simulink model "ba"  (R2022a)
settings: Solver=ode45  StartTime=0.0  StopTime=20  FixedStep=0.001  MaxStep=0.4  RelTol=1e-3  EnableMultiTasking=on
settings Model: ExtModeTrigMode=oneshot  ExtModeArmWhenConnect=off  Creator=liujk  LastModifiedBy=961007prl
settings SolverCC: AlgebraicLoopSolver=TrustRegion
settings DataIOCC: SaveFormat=Array  SignalLoggingSaveFormat=ModelDataLogs  ReturnWorkspaceOutputs=off  SignalLoggingName=sigsOut
settings OptimizationCC: BooleanDataType=off  LifeSpan=inf
settings DebuggingCC: SaveWithParameterizedLinksMsg=none  UnderspecifiedInitializationDetection=Classic  MergeDetectMultiDrivingBlocksExec=none  SignalResolutionControl=TryResolveAllWithWarning  MultiTaskDSMMsg=warning  MultiTaskCondExecSysMsg=none  UnconnectedInputMsg=warning  UnconnectedOutputMsg=warning  UnconnectedLineMsg=warning  StateNameClashWarn=warning  SFUnexpectedBacktrackingDiag=warning  SFNoUnconditionalDefaultTransitionDiag=warning  SFExecutionAtInitializationDiag=none  SFMachineParentedDataDiag=warning  ArithmeticOperatorsInVariantConditions=warning
settings HardwareCC: ProdBitPerPointer=32  ProdBitPerSizeT=32  ProdBitPerPtrDiffT=32  ProdLargestAtomicFloat=None  ProdIntDivRoundTo=Undefined  ProdEndianess=Unspecified  ProdWordSize=32  ProdHWDeviceType=32-bit Generic  TargetUnknown=on
settings ModelReferenceCC: PropagateSignalLabelsOutOfModel=off
settings SFSimCC: SimUseLocalCustomCode=off  CustomCodeUndefinedFunction=UseInterfaceOnly
settings RTWCC: RTWUseLocalCustomCode=off
settings CodeAppCC: StateflowObjectComments=on
settings GRTTargetCC: TargetLangStandard=C89/C90 (ANSI)  CombineOutputUpdateFcns=off  GRTInterface=on
settings ConfigComp: CovMetricSettings=dw  CovSaveCumulativeToWorkspaceVar=on  CovSaveSingleToWorkspaceVar=on  CovExternalEMLEnable=off  CovSFcnEnable=off

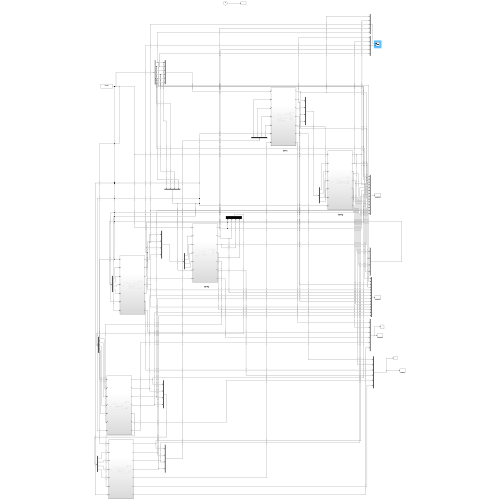
[thumbnail: Simulink's stored preview of the top-level diagram]
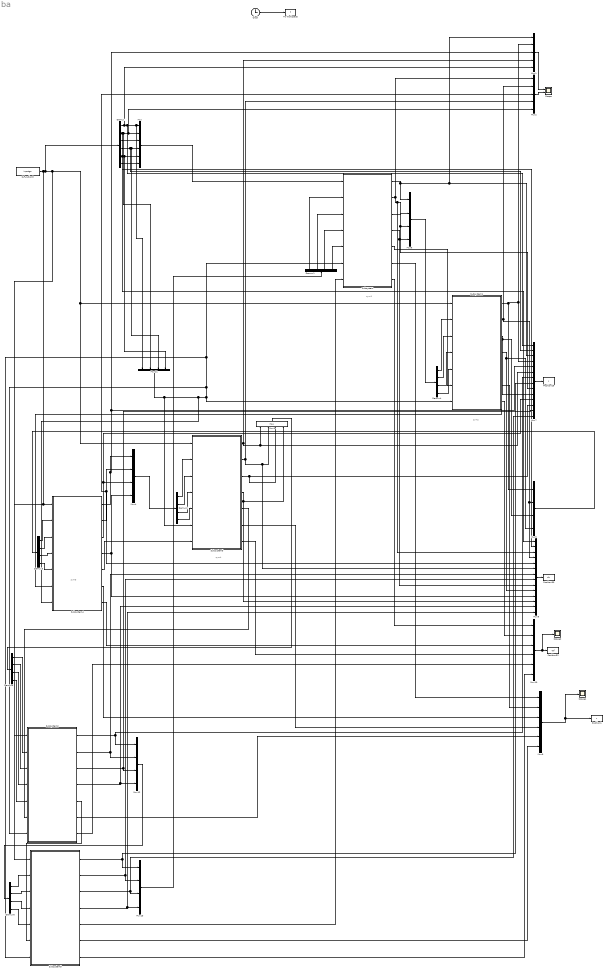
== system ba ==
  note: sym3
  note: sym4
  note: sym2
  note: sym1
  Clock : Clock
  Demux : Demux  Outputs=6
  Demux{1..6} (6 alike) : Demux
  Mux : Mux  Inputs=6
  Mux1 : Mux  Inputs=5
  Mux10 : Mux  Inputs=6
  Mux{3..6,11..13} (7 alike) : Mux
  Mux2 : Mux  Inputs=5
  Mux7 : Mux  Inputs=14
  Mux8 : Mux  Inputs=14
  Mux9 : Mux  Inputs=6
  Position1 : ToWorkspace  VariableName=v  SampleTime=-1
  Position29 : ToWorkspace  VariableName=x  SampleTime=-1
  Position30 : ToWorkspace  VariableName=dx  SampleTime=-1
  Position32 : ToWorkspace  VariableName=Wf  SampleTime=-1
  S-Function3 : S-Function  FunctionName=inputgc  SFunctionDeploymentMode=off  EnableBusSupport=off
  Scope : Scope  NumInputPorts=2
  Scope1 : Scope
  Scope2 : Scope
  Subsystem : Subsystem
  Subsystem1 : Subsystem
  Subsystem2 : Subsystem
  Subsystem3 : Subsystem
  Subsystem4 : Subsystem
  Subsystem5 : Subsystem
  To Workspace : ToWorkspace  VariableName=t  SampleTime=-1
  wires:
  Subsystem/1(Out1) -> Mux6/1, Mux7/3, Mux1/1
  Subsystem/3(Out6) -> Mux7/9, Mux6/3
  Subsystem1/4(Out7) -> Mux8/10, Mux5/4
  Subsystem1/2(Out5) -> Mux5/2, Mux8/4, Mux2/2
  Subsystem4/4(Out7) -> Mux8/11, Mux4/4
  Subsystem4/3(Out6) -> Mux7/11, Mux4/3
  Subsystem4/2(Out5) -> Mux2/3, Mux4/2, Mux8/5
  Subsystem3/1(Out1) -> Mux7/6, Mux3/1, Mux1/4
  Subsystem3/3(Out6) -> Mux3/3, Mux7/12
  S-Function3/1 -> Subsystem5/1(In2), Subsystem3/1(In2), Subsystem1/1(In2), Demux/1, Subsystem2/1(In2), Subsystem4/1(In2)
  Demux/2 -> Mux2/5, Mux/2, Mux11/2, Mux8/1
  Demux/5 -> Mux/5, Mux11/4, Mux8/2
  Subsystem1/7(Out2) -> Mux10/2
  Subsystem/7(Out2) -> Mux10/1
  Demux/6 -> Mux/6
  Demux/4 -> Mux11/3, Mux/4, Mux7/2
  Mux2/1 -> Scope/2
  Mux7/1 -> Position29/1
  Subsystem/4(Out7) -> Mux8/9, Mux6/4
  Demux/3 -> Mux/3
  Subsystem4/7(Out2) -> Mux10/3
  Subsystem4/1(Out1) -> Mux4/1, Mux7/5, Mux1/3
  Mux10/1 -> Scope2/1, Position32/1
  Subsystem1/3(Out6) -> Mux7/10, Mux5/3
  Demux1/1 -> Subsystem/2(In2)
  Demux2/1 -> Subsystem3/2(In1)
  Subsystem3/7(Out2) -> Mux10/4
  Demux2/3 -> Subsystem3/4(In8)
  Demux1/4 -> Subsystem/5(In5)
  Demux3/2 -> Subsystem4/3(In4)
  Demux2/2 -> Subsystem3/3(In7)
  Mux1/1 -> Scope/1
  Clock/1 -> To Workspace/1
  Demux3/4 -> Subsystem4/5(In6)
  Demux3/1 -> Subsystem4/2(In3)
  Subsystem1/1(Out1) -> Mux5/1, Mux7/4, Mux1/2
  Demux3/3 -> Subsystem4/4(In5)
  Mux/1 -> Subsystem/1(In1)
  Demux4/2 -> Subsystem1/3(In4)
  Subsystem/2(Out5) -> Mux8/3, Mux6/2, Mux2/1
  Subsystem3/4(Out7) -> Mux8/12, Mux3/4
  Demux1/2 -> Subsystem/3(In3)
  Mux8/1 -> Position30/1
  Demux1/3 -> Subsystem/4(In4)
  Demux4/3 -> Subsystem1/4(In5)
  Demux4/4 -> Subsystem1/5(In6)
  Demux/1 -> Mux/1, Mux11/1, Mux7/1, Mux1/5
  Demux4/1 -> Subsystem1/2(In3)
  Subsystem3/2(Out5) -> Mux8/6, Mux3/2, Mux2/4
  Demux2/4 -> Subsystem3/5(In9)
  Mux5/1 -> Demux3/1
  Mux11/1 -> Subsystem4/7(In7), Subsystem5/7(In7), Subsystem/6(In6), Subsystem2/7(In7), Subsystem1/7(In7), Subsystem3/6(In10)
  Mux6/1 -> Demux4/1
  Subsystem/5(Out3) -> Subsystem1/6(In1)
  Subsystem1/5(Out3) -> Subsystem4/6(In1)
  Mux9/1 -> Scope1/1, Position1/1
  Subsystem/6(Out4) -> Mux9/1
  Subsystem1/6(Out4) -> Mux9/2
  Subsystem4/6(Out4) -> Mux9/3
  Subsystem3/6(Out4) -> Mux9/4
  Demux5/1 -> Subsystem2/2(In3)
  Demux5/2 -> Subsystem2/3(In4)
  Demux5/3 -> Subsystem2/4(In5)
  Demux5/4 -> Subsystem2/5(In6)
  Subsystem2/3(Out6) -> Mux12/3, Mux7/13
  Subsystem2/4(Out7) -> Mux8/13, Mux12/4
  Subsystem2/1(Out1) -> Mux12/1, Mux7/7
  Subsystem2/2(Out5) -> Mux12/2, Mux8/7
  Subsystem5/2(Out5) -> Mux13/2, Mux8/8
  Subsystem5/3(Out6) -> Mux13/3, Mux7/14
  Subsystem5/4(Out7) -> Mux8/14, Mux13/4
  Subsystem5/1(Out1) -> Mux13/1, Mux7/8
  Demux6/1 -> Subsystem5/2(In3)
  Demux6/2 -> Subsystem5/3(In4)
  Demux6/3 -> Subsystem5/4(In5)
  Demux6/4 -> Subsystem5/5(In6)
  Mux12/1 -> Demux6/1
  Subsystem2/5(Out3) -> Subsystem5/6(In1)
  Subsystem2/6(Out4) -> Mux9/5
  Subsystem5/6(Out4) -> Mux9/6
  Subsystem5/5(Out3) -> Subsystem/7(In7)
  Subsystem4/5(Out3) -> Subsystem3/7(In3)
  Subsystem3/5(Out3) -> Subsystem2/6(In1)
  Mux13/1 -> Demux1/1
  Mux3/1 -> Demux5/1
  Subsystem2/7(Out2) -> Mux10/5
  Subsystem5/7(Out2) -> Mux10/6
  Mux4/1 -> Demux2/1

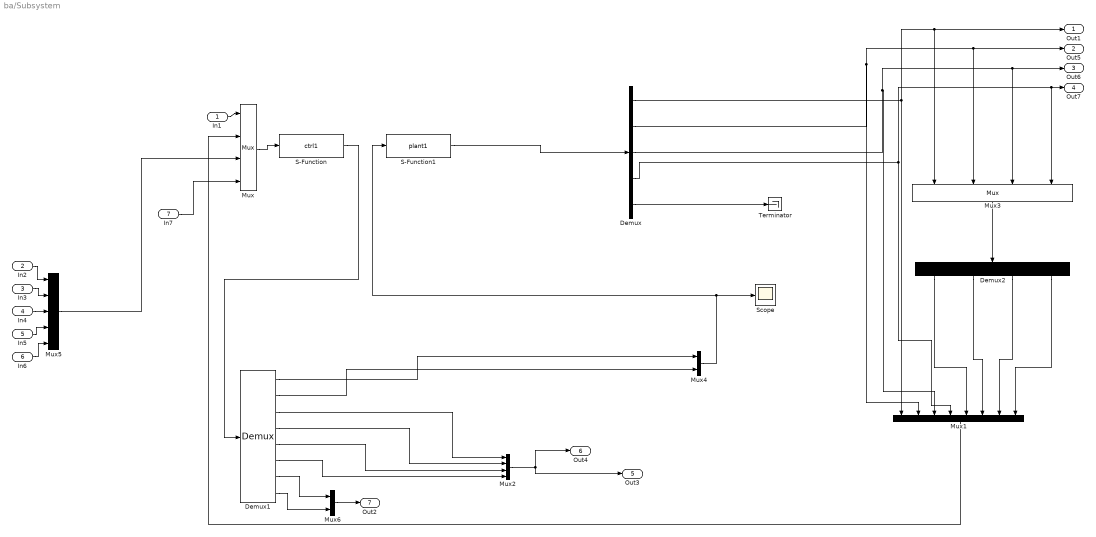
== system ba/Subsystem ==
  In1 : Inport
  In2 : Inport  Port=2
  In3 : Inport  Port=3
  In4 : Inport  Port=4
  In5 : Inport  Port=5
  In6 : Inport  Port=6
  In7 : Inport  Port=7
  Demux : Demux  Outputs=5
  Demux1 : Demux  Outputs=8
  Demux2 : Demux
  Mux : Mux
  Mux1 : Mux  Inputs=8
  Mux2 : Mux
  Mux3 : Mux
  Mux4 : Mux  Inputs=2
  Mux5 : Mux  Inputs=5
  Mux6 : Mux  Inputs=2
  S-Function : S-Function  FunctionName=ctrl1  SFunctionDeploymentMode=off  EnableBusSupport=off
  S-Function1 : S-Function  FunctionName=plant1  SFunctionDeploymentMode=off  EnableBusSupport=off
  Scope : Scope
  Terminator : Terminator
  Out1 : Outport
  Out5 : Outport  Port=2
  Out6 : Outport  Port=3
  Out7 : Outport  Port=4
  Out3 : Outport  Port=5
  Out4 : Outport  Port=6
  Out2 : Outport  Port=7
  wires:
  Mux/1 -> S-Function/1
  In1/1 -> Mux/1
  S-Function/1 -> Demux1/1
  Demux1/1 -> Mux4/1
  Mux4/1 -> S-Function1/1, Scope/1
  S-Function1/1 -> Demux/1
  Demux/5 -> Terminator/1
  Demux1/2 -> Mux4/2
  In2/1 -> Mux5/1
  In3/1 -> Mux5/2
  In4/1 -> Mux5/3
  In5/1 -> Mux5/4
  In6/1 -> Mux5/5
  Mux5/1 -> Mux/3
  Mux1/1 -> Mux/2
  Demux/2 -> Mux3/2, Out5/1, Mux1/2
  Demux2/3 -> Mux1/7
  Demux2/4 -> Mux1/8
  Demux2/2 -> Mux1/6
  Demux/3 -> Mux3/3, Out6/1, Mux1/3
  Demux/4 -> Mux3/4, Out7/1, Mux1/4
  Demux/1 -> Mux3/1, Out1/1, Mux1/1
  Demux2/1 -> Mux1/5
  Demux1/3 -> Mux2/1
  Demux1/4 -> Mux2/2
  Demux1/5 -> Mux2/3
  Demux1/6 -> Mux2/4
  Mux2/1 -> Out3/1, Out4/1
  In7/1 -> Mux/4
  Demux1/7 -> Mux6/1
  Demux1/8 -> Mux6/2
  Mux6/1 -> Out2/1
  Mux3/1 -> Demux2/1

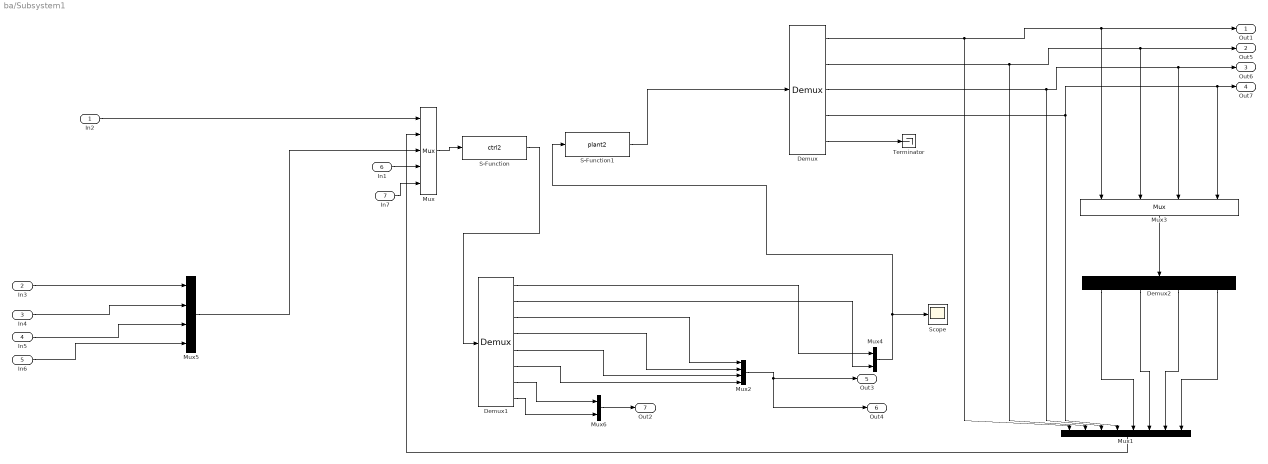
== system ba/Subsystem1 ==
  In2 : Inport
  In3 : Inport  Port=2
  In4 : Inport  Port=3
  In5 : Inport  Port=4
  In6 : Inport  Port=5
  In1 : Inport  Port=6
  In7 : Inport  Port=7
  Demux : Demux  Outputs=5
  Demux1 : Demux  Outputs=8
  Demux2 : Demux
  Mux : Mux  Inputs=5
  Mux1 : Mux  Inputs=8
  Mux2 : Mux
  Mux3 : Mux
  Mux4 : Mux  Inputs=2
  Mux5 : Mux
  Mux6 : Mux  Inputs=2
  S-Function : S-Function  FunctionName=ctrl2  SFunctionDeploymentMode=off  EnableBusSupport=off
  S-Function1 : S-Function  FunctionName=plant2  SFunctionDeploymentMode=off  EnableBusSupport=off
  Scope : Scope
  Terminator : Terminator
  Out1 : Outport
  Out5 : Outport  Port=2
  Out6 : Outport  Port=3
  Out7 : Outport  Port=4
  Out3 : Outport  Port=5
  Out4 : Outport  Port=6
  Out2 : Outport  Port=7
  wires:
  Mux/1 -> S-Function/1
  S-Function/1 -> Demux1/1
  Demux1/1 -> Mux4/1
  S-Function1/1 -> Demux/1
  Demux/5 -> Terminator/1
  In3/1 -> Mux5/1
  In4/1 -> Mux5/2
  In5/1 -> Mux5/3
  In6/1 -> Mux5/4
  In2/1 -> Mux/1
  Mux5/1 -> Mux/3
  Mux4/1 -> S-Function1/1, Scope/1
  Demux2/3 -> Mux1/7
  Demux/1 -> Out1/1, Mux3/1, Mux1/1
  Demux2/2 -> Mux1/6
  Mux1/1 -> Mux/2
  Demux2/1 -> Mux1/5
  Demux/2 -> Out5/1, Mux3/2, Mux1/2
  Demux2/4 -> Mux1/8
  Demux/3 -> Out6/1, Mux3/3, Mux1/3
  Demux/4 -> Out7/1, Mux3/4, Mux1/4
  Mux3/1 -> Demux2/1
  Demux1/2 -> Mux4/2
  Demux1/4 -> Mux2/2
  Mux2/1 -> Out3/1, Out4/1
  Demux1/3 -> Mux2/1
  Demux1/5 -> Mux2/3
  Demux1/6 -> Mux2/4
  In1/1 -> Mux/4
  In7/1 -> Mux/5
  Demux1/7 -> Mux6/1
  Demux1/8 -> Mux6/2
  Mux6/1 -> Out2/1

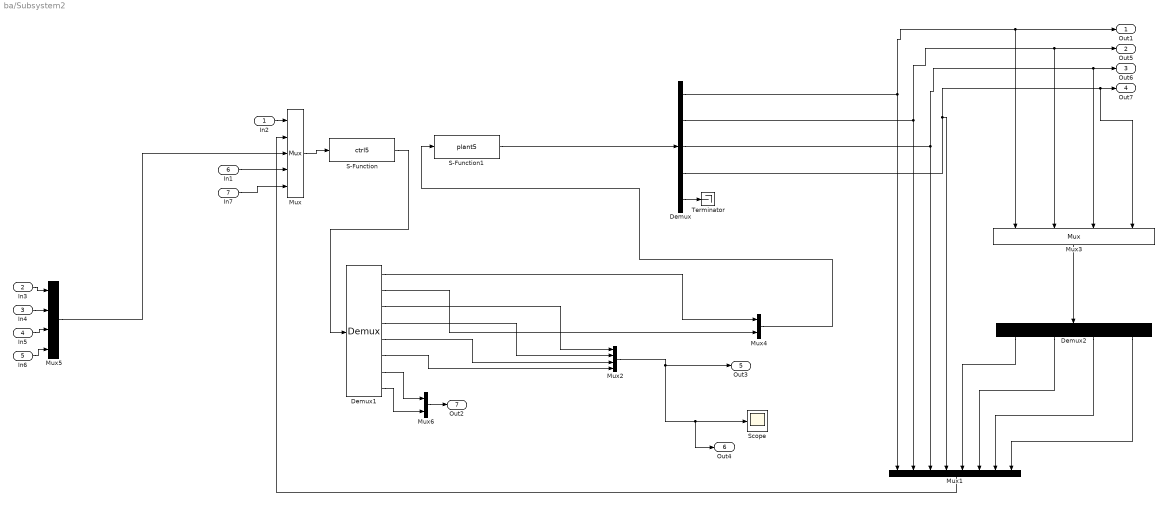
== system ba/Subsystem2 ==
  In2 : Inport
  In3 : Inport  Port=2
  In4 : Inport  Port=3
  In5 : Inport  Port=4
  In6 : Inport  Port=5
  In1 : Inport  Port=6
  In7 : Inport  Port=7
  Demux : Demux  Outputs=5
  Demux1 : Demux  Outputs=8
  Demux2 : Demux
  Mux : Mux  Inputs=5
  Mux1 : Mux  Inputs=8
  Mux2 : Mux
  Mux3 : Mux
  Mux4 : Mux  Inputs=2
  Mux5 : Mux
  Mux6 : Mux  Inputs=2
  S-Function : S-Function  FunctionName=ctrl5  SFunctionDeploymentMode=off  EnableBusSupport=off
  S-Function1 : S-Function  FunctionName=plant5  SFunctionDeploymentMode=off  EnableBusSupport=off
  Scope : Scope
  Terminator : Terminator
  Out1 : Outport
  Out5 : Outport  Port=2
  Out6 : Outport  Port=3
  Out7 : Outport  Port=4
  Out3 : Outport  Port=5
  Out4 : Outport  Port=6
  Out2 : Outport  Port=7
  wires:
  Mux/1 -> S-Function/1
  S-Function/1 -> Demux1/1
  S-Function1/1 -> Demux/1
  Demux/5 -> Terminator/1
  In3/1 -> Mux5/1
  In4/1 -> Mux5/2
  In5/1 -> Mux5/3
  In6/1 -> Mux5/4
  In2/1 -> Mux/1
  Mux5/1 -> Mux/3
  Mux4/1 -> S-Function1/1
  Mux1/1 -> Mux/2
  Demux1/1 -> Mux4/1
  Demux1/2 -> Mux4/2
  Demux/2 -> Out5/1, Mux3/2, Mux1/2
  Demux2/3 -> Mux1/7
  Demux2/4 -> Mux1/8
  Demux2/2 -> Mux1/6
  Demux/3 -> Out6/1, Mux3/3, Mux1/3
  Demux/4 -> Out7/1, Mux3/4, Mux1/4
  Demux/1 -> Mux3/1, Out1/1, Mux1/1
  Demux2/1 -> Mux1/5
  Mux3/1 -> Demux2/1
  Demux1/4 -> Mux2/2
  Mux2/1 -> Out3/1, Out4/1, Scope/1
  Demux1/3 -> Mux2/1
  Demux1/5 -> Mux2/3
  Demux1/6 -> Mux2/4
  In1/1 -> Mux/4
  In7/1 -> Mux/5
  Demux1/7 -> Mux6/1
  Demux1/8 -> Mux6/2
  Mux6/1 -> Out2/1

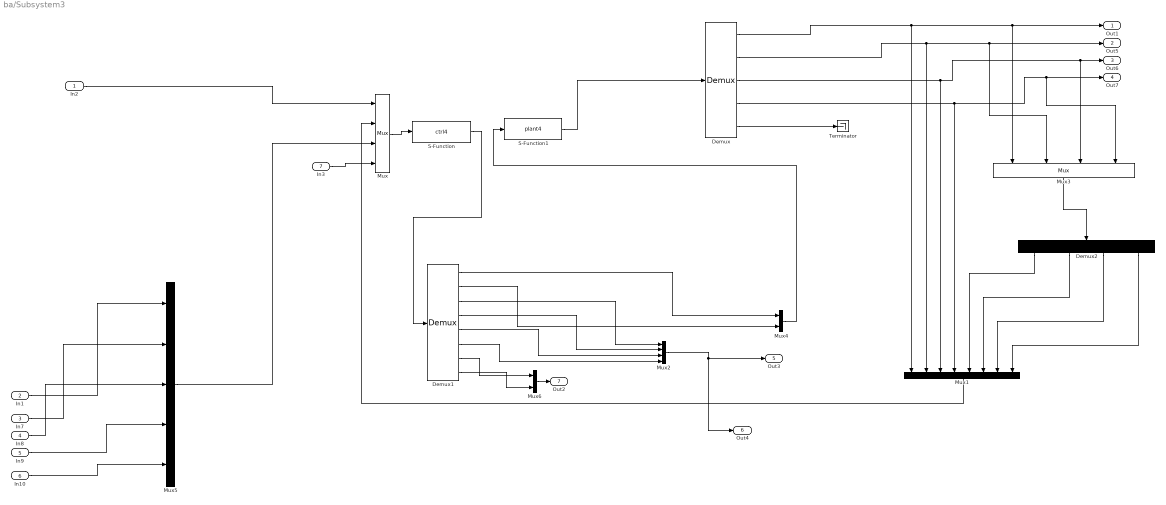
== system ba/Subsystem3 ==
  In2 : Inport
  In1 : Inport  Port=2
  In7 : Inport  Port=3
  In8 : Inport  Port=4
  In9 : Inport  Port=5
  In10 : Inport  Port=6
  In3 : Inport  Port=7
  Demux : Demux  Outputs=5
  Demux1 : Demux  Outputs=8
  Demux2 : Demux
  Mux : Mux
  Mux1 : Mux  Inputs=8
  Mux2 : Mux
  Mux3 : Mux
  Mux4 : Mux  Inputs=2
  Mux5 : Mux  Inputs=5
  Mux6 : Mux  Inputs=2
  S-Function : S-Function  FunctionName=ctrl4  SFunctionDeploymentMode=off  EnableBusSupport=off
  S-Function1 : S-Function  FunctionName=plant4  SFunctionDeploymentMode=off  EnableBusSupport=off
  Terminator : Terminator
  Out1 : Outport
  Out5 : Outport  Port=2
  Out6 : Outport  Port=3
  Out7 : Outport  Port=4
  Out3 : Outport  Port=5
  Out4 : Outport  Port=6
  Out2 : Outport  Port=7
  wires:
  Mux/1 -> S-Function/1
  S-Function/1 -> Demux1/1
  Demux1/1 -> Mux4/1
  S-Function1/1 -> Demux/1
  Demux/5 -> Terminator/1
  In2/1 -> Mux/1
  Mux5/1 -> Mux/3
  Mux4/1 -> S-Function1/1
  In1/1 -> Mux5/1
  In7/1 -> Mux5/2
  In8/1 -> Mux5/3
  In9/1 -> Mux5/4
  In10/1 -> Mux5/5
  Mux1/1 -> Mux/2
  Demux/2 -> Mux3/2, Out5/1, Mux1/2
  Demux2/3 -> Mux1/7
  Demux2/4 -> Mux1/8
  Demux2/2 -> Mux1/6
  Demux/3 -> Mux1/3, Mux3/3, Out6/1
  Demux/4 -> Mux1/4, Mux3/4, Out7/1
  Demux/1 -> Mux1/1, Mux3/1, Out1/1
  Demux2/1 -> Mux1/5
  Demux1/2 -> Mux4/2
  Demux1/4 -> Mux2/2
  Demux1/3 -> Mux2/1
  Demux1/5 -> Mux2/3
  Demux1/6 -> Mux2/4
  In3/1 -> Mux/4
  Mux2/1 -> Out3/1, Out4/1
  Demux1/7 -> Mux6/1
  Demux1/8 -> Mux6/2
  Mux6/1 -> Out2/1
  Mux3/1 -> Demux2/1

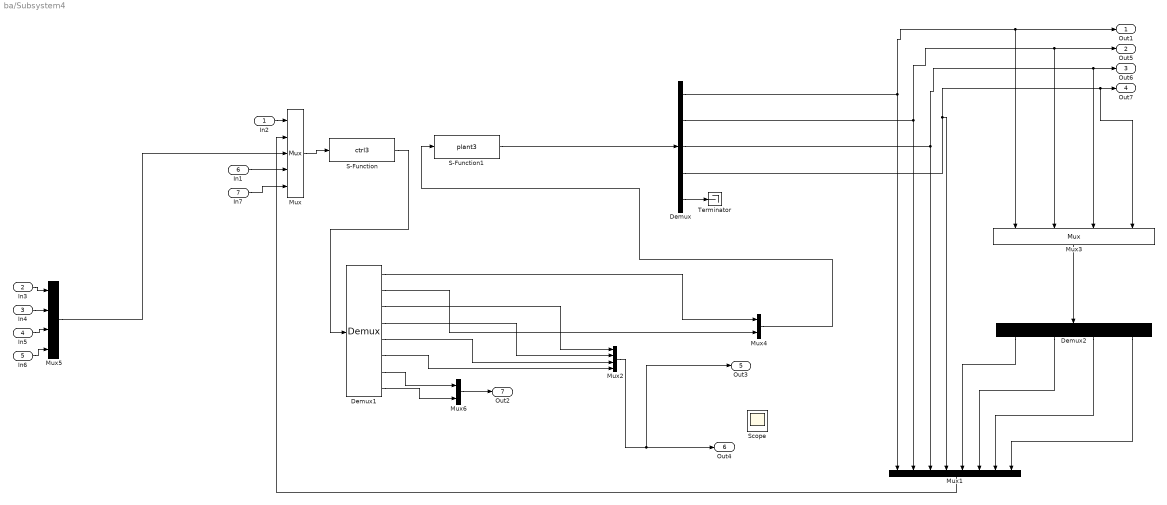
== system ba/Subsystem4 ==
  In2 : Inport
  In3 : Inport  Port=2
  In4 : Inport  Port=3
  In5 : Inport  Port=4
  In6 : Inport  Port=5
  In1 : Inport  Port=6
  In7 : Inport  Port=7
  Demux : Demux  Outputs=5
  Demux1 : Demux  Outputs=8
  Demux2 : Demux
  Mux : Mux  Inputs=5
  Mux1 : Mux  Inputs=8
  Mux2 : Mux
  Mux3 : Mux
  Mux4 : Mux  Inputs=2
  Mux5 : Mux
  Mux6 : Mux  Inputs=2
  S-Function : S-Function  FunctionName=ctrl3  SFunctionDeploymentMode=off  EnableBusSupport=off
  S-Function1 : S-Function  FunctionName=plant3  SFunctionDeploymentMode=off  EnableBusSupport=off
  Scope : Scope
  Terminator : Terminator
  Out1 : Outport
  Out5 : Outport  Port=2
  Out6 : Outport  Port=3
  Out7 : Outport  Port=4
  Out3 : Outport  Port=5
  Out4 : Outport  Port=6
  Out2 : Outport  Port=7
  wires:
  Mux/1 -> S-Function/1
  S-Function/1 -> Demux1/1
  S-Function1/1 -> Demux/1
  Demux/5 -> Terminator/1
  In3/1 -> Mux5/1
  In4/1 -> Mux5/2
  In5/1 -> Mux5/3
  In6/1 -> Mux5/4
  In2/1 -> Mux/1
  Mux5/1 -> Mux/3
  Mux4/1 -> S-Function1/1
  Mux1/1 -> Mux/2
  Demux1/1 -> Mux4/1
  Demux1/2 -> Mux4/2
  Demux/2 -> Out5/1, Mux3/2, Mux1/2
  Demux2/3 -> Mux1/7
  Demux2/4 -> Mux1/8
  Demux2/2 -> Mux1/6
  Demux/3 -> Out6/1, Mux3/3, Mux1/3
  Demux/4 -> Out7/1, Mux3/4, Mux1/4
  Demux/1 -> Mux3/1, Out1/1, Mux1/1
  Demux2/1 -> Mux1/5
  Mux3/1 -> Demux2/1
  Demux1/4 -> Mux2/2
  Mux2/1 -> Out3/1, Out4/1
  Demux1/3 -> Mux2/1
  Demux1/5 -> Mux2/3
  Demux1/6 -> Mux2/4
  In1/1 -> Mux/4
  In7/1 -> Mux/5
  Demux1/7 -> Mux6/1
  Demux1/8 -> Mux6/2
  Mux6/1 -> Out2/1

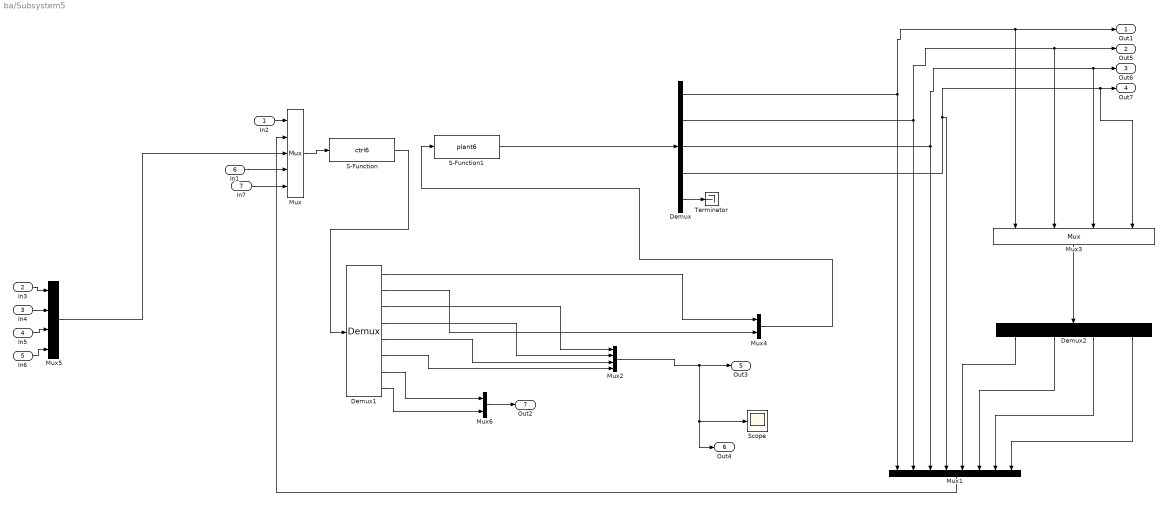
== system ba/Subsystem5 ==
  In2 : Inport
  In3 : Inport  Port=2
  In4 : Inport  Port=3
  In5 : Inport  Port=4
  In6 : Inport  Port=5
  In1 : Inport  Port=6
  In7 : Inport  Port=7
  Demux : Demux  Outputs=5
  Demux1 : Demux  Outputs=8
  Demux2 : Demux
  Mux : Mux  Inputs=5
  Mux1 : Mux  Inputs=8
  Mux2 : Mux
  Mux3 : Mux
  Mux4 : Mux  Inputs=2
  Mux5 : Mux
  Mux6 : Mux  Inputs=2
  S-Function : S-Function  FunctionName=ctrl6  SFunctionDeploymentMode=off  EnableBusSupport=off
  S-Function1 : S-Function  FunctionName=plant6  SFunctionDeploymentMode=off  EnableBusSupport=off
  Scope : Scope
  Terminator : Terminator
  Out1 : Outport
  Out5 : Outport  Port=2
  Out6 : Outport  Port=3
  Out7 : Outport  Port=4
  Out3 : Outport  Port=5
  Out4 : Outport  Port=6
  Out2 : Outport  Port=7
  wires:
  Mux/1 -> S-Function/1
  S-Function/1 -> Demux1/1
  S-Function1/1 -> Demux/1
  Demux/5 -> Terminator/1
  In3/1 -> Mux5/1
  In4/1 -> Mux5/2
  In5/1 -> Mux5/3
  In6/1 -> Mux5/4
  In2/1 -> Mux/1
  Mux5/1 -> Mux/3
  Mux4/1 -> S-Function1/1
  Mux1/1 -> Mux/2
  Demux1/1 -> Mux4/1
  Demux1/2 -> Mux4/2
  Demux/2 -> Out5/1, Mux3/2, Mux1/2
  Demux2/3 -> Mux1/7
  Demux2/4 -> Mux1/8
  Demux2/2 -> Mux1/6
  Demux/3 -> Out6/1, Mux3/3, Mux1/3
  Demux/4 -> Out7/1, Mux3/4, Mux1/4
  Demux/1 -> Mux3/1, Out1/1, Mux1/1
  Demux2/1 -> Mux1/5
  Mux3/1 -> Demux2/1
  Demux1/4 -> Mux2/2
  Mux2/1 -> Scope/1, Out4/1, Out3/1
  Demux1/3 -> Mux2/1
  Demux1/5 -> Mux2/3
  Demux1/6 -> Mux2/4
  In1/1 -> Mux/4
  In7/1 -> Mux/5
  Demux1/7 -> Mux6/1
  Demux1/8 -> Mux6/2
  Mux6/1 -> Out2/1
